simulink model "offline_model"  (R2024a)
settings: Solver=VariableStepAuto  StartTime=0.0  StopTime=60  RelTol=1e-3
values from neighbouring files (symbols this model uses):
  fs = 250    [ssvep_gen_MATLAB.m]
undefined symbols (not defined in the file or in its folder): fdesignblkfcn, gcbh
libraries: dspxfrm3 x1, dspstat3 x1, dspsigops x1, dspnetwork x1
settings Model: Creator=Hristo Marinov  LastModifiedBy=Hristo Marinov

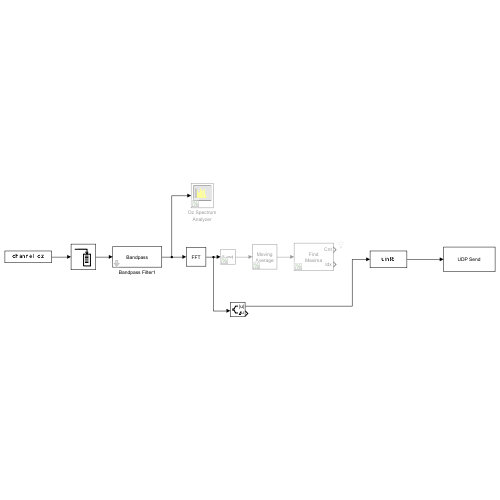
[thumbnail: Simulink's stored preview of the top-level diagram]
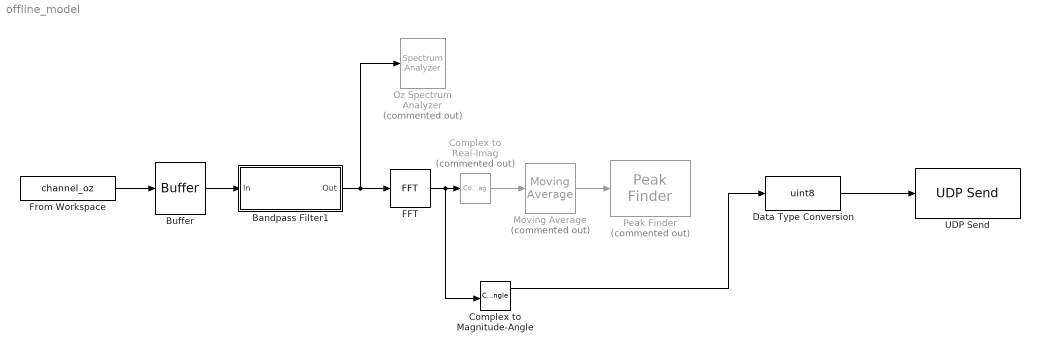
== system offline_model ==
  Bandpass Filter1 : Subsystem  DialogController=fdesignblkfcn  InitFcn=fdesignblkfcn(gcbh, {'InitFcn'});  mask(Bandpass Filter){}
      mask help: Design a bandpass filter
      settings: CopyFcn=fdesignblkfcn(gcbh, {'CopyFcn'});
      mask Help: helpview(mapfilelocation('dsp'), 'dspbandpassfilter');
      mask Display: disp('Bandpass');
  Buffer : Buffer  N=1000  OutputFrames=off
  Complex to Magnitude-Angle : ComplexToMagnitudeAngle
  Complex to Real-Imag : ComplexToRealImag  Commented=on  Output=Real
  Data Type Conversion : DataTypeConversion  OutDataTypeStr=uint8  SaturateOnIntegerOverflow=off  RndMeth=Floor
  FFT : dspxfrm3/FFT  FFTImplementation=Auto  CompMethod=Table lookup  TableOpt=NEW  TableOptActive=Speed  BitRevOrder=off  Normalize=off  InheritFFTLength=on  FFTLength=64  WrapInput=on  roundingMode=Ceiling  overflowMode=off  firstCoeffDataTypeStr=Inherit: Same word length as input  firstCoeffLastDataTypeStr=Inherit: Same word length as input  outputMin=[]  outputMax=[]
  From Workspace : FromWorkspace  VariableName=channel_oz  SampleTime=1/fs
  Moving Average : dspstat3/Moving Average  Commented=on  Method=Exponential weighting  ForgettingFactorPort=off  SpecifyWindowLength=on  WindowLength=4  OverlapLength=3  AllowArbitraryInputLength=off  ForgettingFactor=0  SimulateUsing=Interpreted execution
  Oz Spectrum Analyzer : SpectrumAnalyzer  Commented=on  WindowPosition=[86.000000,34.000000,958.000000,1000.000000,]  ScopeFrameLocation=window  ViewType=Spectrum and spectrogram  Method=Welch  PlotAsTwoSidedSpectrum=off  FrequencyResolutionMethod=Window length  Span=125  CenterFrequency=62.5  StartFrequency=0  StopFrequency=125  AveragingMethod=Exponential  ForgettingFactor=0  TimeSpanSource=Property  TimeSpan=60  YLimits=[-111.54212863,90.55320398]  ColorLimits=[-111.54212863,90.55320398]
  Peak Finder : dspsigops/Peak Finder  Commented=on  polarity=Maxima  indexBase=Zero  outputIdx=on  outputVal=off  maxPeaks=3  NoiseDistinguish=off  thresh=0  roundingMode=Floor  overflowMode=off
      settings: allowOverrides=off
  UDP Send : dspnetwork/UDP Send  remoteURL='127.0.0.1'  remotePort=5005  localURL='0.0.0.0'  localPortSource=Automatically determine  localPort=-1  sendBufferSize=8192  sampletime=-1  blockPlatform=[]  separateLengthPort=0
      settings: LibrarySourceBlock=dspsnks4/UDP Send
  wires:
  Bandpass Filter1/1(Out) -> Oz Spectrum Analyzer/1, FFT/1
  From Workspace/1 -> Buffer/1
  Data Type Conversion/1 -> UDP Send/1
  FFT/1 -> Complex to Magnitude-Angle/1, Complex to Real-Imag/1
  Moving Average/1 -> Peak Finder/1
  Complex to Real-Imag/1 -> Moving Average/1
  Buffer/1 -> Bandpass Filter1/1(In)
  Complex to Magnitude-Angle/1 -> Data Type Conversion/1

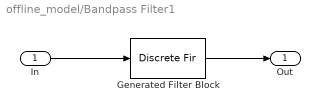
== system offline_model/Bandpass Filter1 ==
  In : Inport
  Generated Filter Block : DiscreteFir  Tag=BlockMethodSubSystem  Coefficients=[-0.000426262391371108704 9.67719260516699165e-05 -7.3223551323464846e-06 -0.000159620452654756498 -0.000356064632503387188 -0.000584942555056474169 -0.000819977007863703883 -0.00101896180508245912 -0.00112780073150509693 -0.0010904347816387658 -0.000861646475751319833 -0.000420869516592750929 0.000217341233221154945 0.000998221865196268236 0.00183015718617887094 0.00259585009352567442 0.00317109634670075359 0.00344686782575220159 0.00335159389783438273 0.00286781781899178752 0.00204025748527656824 0.000971852127560903726 -0.000191289671027485643 -0.00128483321858502311 -0.00215530831745061905 -0.00268877582668294694 -0.00283198196080375201 -0.00260243665892021013 -0.00208394123055433535 -0.00140915819500849284 -0.000731644603052826795 -0.000194217690398635614 0.000100728489832094633 0.000111438758339274852 -0.000136331986042842381 -0.000555737231142244608 -0.00102442560520670596 -0.00140616190319969099 -0.00159111898002007191 -0.00151586776883213203 -0.00117806859682025706 -0.000638016748052914681 -3.2204827010274508e-06 0.000598093401315346251 0.00104798544109993455 0.00126627117031328606 0.00122933577855054306 0.000975004791883010897 0.000592971409791488691 0.000202008317269161458 -7.94910412151391863e-05 -0.000163397478043984925 -1.36295437819857617e-05 0.000344493434996724103 0.000830684385452651938 0.00132939587377283548 0.00171887879004453833 0.0019014551578723489 0.00182852242303469512 0.00151282688344080716 0.00102596160601962244 0.000480495206059551041 2.09577320117238857e-06 -0.000302372366356881488 -0.000371815560615083548 -0.000206993263427584666 0.000129479698597615355 0.000528372677185778958 0.000861649752273612791 0.00101523179561079134 0.000918329241447135135 0.000563575431311902179 8.45606748774664655e-06 -0.000636110522660805213 -0.00123421121956375068 -0.00165905271089605497 -0.00182442532330057833 -0.00170774754438343473 -0.00135656830090702786 -0.0008771927302180277 -0.000407723665371088656 -8.32528444012840379e-05 -6.67241551999882795e-07 -0.00019294387067110875 -0.000618955803950309779 -0.00117285870791726489 -0.00170981485118795458 -0.00208279597118924548 -0.0021801307490026435 -0.00195527669038719808 -0.00144006302621936316 -0.000738565769353007246 -1.75111845054039163e-06 0.000609892747322387033 0.000967527782794247969 0.00100720651122678667 0.000747546814900256515 0.000285993926920607446 -0.000224869300378212935 -0.000616206658784346087 -0.000746393774788387996 -0.000538931048631869237 -3.88359469951969189e-06 0.00076205250175562407 0.00159817108054648334 0.00231939974890195758 0.00276266957602670305 0.0028296987595557415 0.00251272360917145299 0.0018985698031324025 0.00114827217923365449 0.000456384487303368555 1.86333088087149633e-06 -9.87838626993313846e-05 0.000177003812423875094 0.000749681171947524884 0.00145627672489359985 0.00209043404431733144 0.002455117136998081 0.00241382769212259655 0.00192802683657232986 0.00106951988893315788 5.25459979922084294e-06 -0.00104323592631712608 -0.00185486946640072217 -0.00226570951296400187 -0.00221176465075508455 -0.00174749070781871595 -0.00103349636159760197 -0.000297145654369973316 0.000225587046408870203 0.000351347734056225265 -1.04694100924397692e-06 -0.000786711684843220162 -0.00184237863076907476 -0.00292539839693066114 -0.0037738052702424806 -0.00417343705279251114 -0.00401393265622260794 -0.00331975414366574625 -0.00224705512492552042 -0.00104644929860546747 -8.99581594550967587e-07 0.000646700813578191197 0.000757012208541265686 0.000332304157858173265 -0.000480518512623423944 -0.0014252137509366109 -0.00220006165740035996 -0.00253555643452365665 -0.00226554208902656059 -0.00137404972262697499 -3.91537063615115771e-06 0.00157482448105955618 0.00303065216548627789 0.00405339923318980781 0.0044343910030460636 0.00412183260801970291 0.00323763626531589285 0.00204936576747554106 0.000904309679494584681 0.000140689516804746805 -5.98605091486901767e-07 0.000558010426980191823 0.00170593200083640588 0.00316711394371623585 0.00456674520724026801 ...(+8207 chars)]  InputProcessing=Columns as channels (frame based)
  Out : Outport
  wires:
  In/1 -> Generated Filter Block/1
  Generated Filter Block/1 -> Out/1
